simulink model "SS_F16_Block"  (Simulink 10.0)
settings: Solver=ode5  StartTime=0.0  StopTime=200  FixedStep=deltaT  RelTol=1e-3  EnableMultiTasking=on
values from neighbouring files (symbols this model uses):
  trim_control = [xu(2);xu(4);xu(5)]    [trim_F16.m]
  trim_thrust = xu(13)    [trim_F16.m]
undefined symbols (not defined in the file or in its folder): A, B, C, D, DisAil_1, DisAil_2, DisAil_3, DisEle_1, DisEle_2, DisEle_3, DisRud_1, DisRud_2, DisRud_3, thrust
settings Model: Creator=russ1110  LastModifiedBy=asmialek  ExtModeAutoUpdateStatusClock=off
settings DataIOCC: LimitDataPoints=on  SignalLoggingName=sigsOut
settings OptimizationCC: BooleanDataType=off  LifeSpan=auto
settings DebuggingCC: SaveWithParameterizedLinksMsg=none  SignalResolutionControl=TryResolveAllWithWarning  MultiTaskDSMMsg=warning  MultiTaskCondExecSysMsg=none  SFUnexpectedBacktrackingDiag=error  SFNoUnconditionalDefaultTransitionDiag=error  SFExecutionAtInitializationDiag=warning
settings HardwareCC: TargetUnknown=on
settings ConfigComp: CovExternalEMLEnable=off

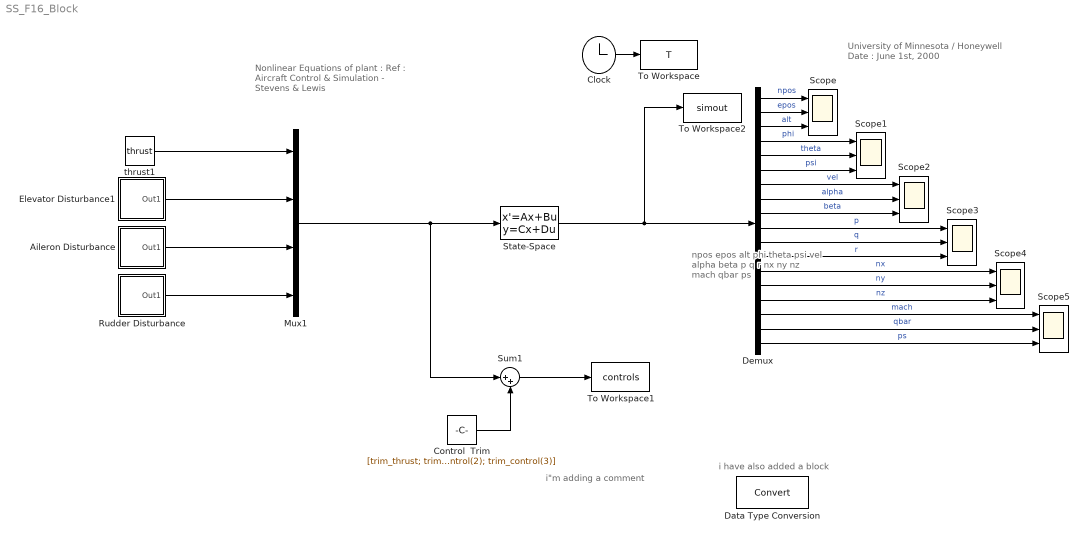
== system SS_F16_Block ==
  note: i have also added a block
  note: i"m adding a comment
  note: npos
      | epos
      | alt
      | phi
      | theta
      | psi
      | vel
      | alpha
      | beta
      | p
      | q
      | r
      | nx
      | ny
      | nz
      | mach
      | qbar
      | ps
  note: University of Minnesota / Honeywell
      | Date : June 1st, 2000
  note: Nonlinear Equations of plant :
      | Ref : Aircraft Control & Simulation
      | - Stevens & Lewis
  Aileron Disturbance : Subsystem
  Clock : Clock
      settings: Decimation=50
  Control  Trim : Constant  Value=[trim_thrust; trim_control(1); trim_control(2); trim_control(3)]
  Data Type Conversion : DataTypeConversion
  Demux : Demux  Outputs=18
  Elevator Disturbance1 : Subsystem
  Mux1 : Mux
  Rudder Disturbance : Subsystem
  Scope{,1..5} (6 alike) : Scope  NumInputPorts=3
  State-Space : StateSpace  A=A  B=B  C=C  D=D  InitialCondition=0
  Sum1 : Sum  Inputs=|++  SaturateOnIntegerOverflow=on  InputSameDT=on  OutDataTypeStr=Inherit: Same as first input
  To Workspace : ToWorkspace  VariableName=T  SampleTime=-1
      settings: Decimation=100
  To Workspace1 : ToWorkspace  VariableName=controls  SampleTime=-1
      settings: Decimation=100
  To Workspace2 : ToWorkspace  VariableName=simout  SampleTime=-1
      settings: Decimation=100
  thrust1 : Constant  Value=thrust  VectorParams1D=off
  wires:
  Clock/1 -> To Workspace/1
  Demux/1 -> Scope/1  "npos"
  Demux/2 -> Scope/2  "epos"
  Demux/3 -> Scope/3  "alt"
  Demux/5 -> Scope1/2  "theta"
  Demux/6 -> Scope1/3  "psi"
  Demux/7 -> Scope2/1  "vel"
  Demux/8 -> Scope2/2  "alpha"
  Demux/9 -> Scope2/3  "beta"
  Demux/10 -> Scope3/1  "p"
  Demux/11 -> Scope3/2  "q"
  Demux/12 -> Scope3/3  "r"
  Demux/13 -> Scope4/1  "nx"
  Demux/14 -> Scope4/2  "ny"
  Demux/15 -> Scope4/3  "nz"
  Demux/4 -> Scope1/1  "phi"
  Demux/16 -> Scope5/1  "mach"
  Demux/17 -> Scope5/2  "qbar"
  Demux/18 -> Scope5/3  "ps"
  Control  Trim/1 -> Sum1/2
  Mux1/1 -> Sum1/1, State-Space/1
  State-Space/1 -> Demux/1, To Workspace2/1
  Elevator Disturbance1/1(Out1) -> Mux1/2
  Aileron Disturbance/1(Out1) -> Mux1/3
  thrust1/1 -> Mux1/1
  Rudder Disturbance/1(Out1) -> Mux1/4
  Sum1/1 -> To Workspace1/1

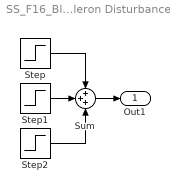
== system SS_F16_Block/Aileron Disturbance ==
  Step : Step  After=DisAil_1  SampleTime=0
  Step1 : Step  Time=3  After=DisAil_2  SampleTime=0
  Step2 : Step  Time=5  After=DisAil_3  SampleTime=0
  Sum : Sum  Inputs=+++  SaturateOnIntegerOverflow=on  InputSameDT=on  OutDataTypeStr=Inherit: Same as first input
  Out1 : Outport  VectorParamsAs1DForOutWhenUnconnected=off
  wires:
  Step1/1 -> Sum/2
  Step/1 -> Sum/1
  Step2/1 -> Sum/3
  Sum/1 -> Out1/1

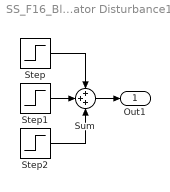
== system SS_F16_Block/Elevator Disturbance1 ==
  Step : Step  After=DisEle_1  SampleTime=0
  Step1 : Step  Time=3  After=DisEle_2  SampleTime=0
  Step2 : Step  Time=5  After=DisEle_3  SampleTime=0
  Sum : Sum  Inputs=+++  SaturateOnIntegerOverflow=on  InputSameDT=on  OutDataTypeStr=Inherit: Same as first input
  Out1 : Outport  VectorParamsAs1DForOutWhenUnconnected=off
  wires:
  Step1/1 -> Sum/2
  Step/1 -> Sum/1
  Step2/1 -> Sum/3
  Sum/1 -> Out1/1

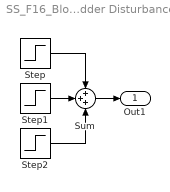
== system SS_F16_Block/Rudder Disturbance ==
  Step : Step  After=DisRud_1  SampleTime=0
  Step1 : Step  Time=1.5  After=DisRud_2  SampleTime=0
  Step2 : Step  Time=2  After=DisRud_3  SampleTime=0
  Sum : Sum  Inputs=+++  SaturateOnIntegerOverflow=on  InputSameDT=on  OutDataTypeStr=Inherit: Same as first input
  Out1 : Outport  VectorParamsAs1DForOutWhenUnconnected=off
  wires:
  Step1/1 -> Sum/2
  Step/1 -> Sum/1
  Step2/1 -> Sum/3
  Sum/1 -> Out1/1
